simulink model "prob3"  (R2020b)
settings: Solver=ode45  StartTime=0.0  StopTime=10.0  RelTol=1e-3
undefined symbols (not defined in the file): b, m
settings Model: Creator=shridhar  LastModifiedBy=shridhar

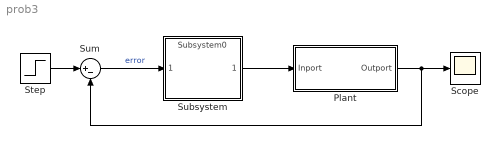
== system prob3 ==
  Plant : Subsystem
  Scope : Scope
  Step : Step  Time=0  After=u  SampleTime=0
  Subsystem : ModelReference  ModelNameDialog=Subsystem0  SimulationMode=Normal  ModelReferenceVersion=1.2
  Sum : Sum  Inputs=|+-
  wires:
  Plant/1(Outport) -> Scope/1, Sum/2
  Step/1 -> Sum/1
  Sum/1 -> Subsystem/1  "error"
  Subsystem/1 -> Plant/1(Inport)

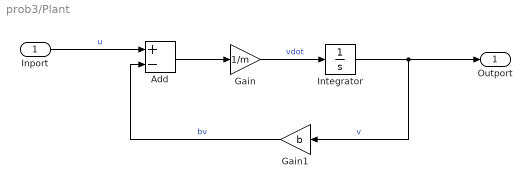
== system prob3/Plant ==
  Inport : Inport
  Add : Sum  Inputs=+-
  Gain : Gain  Gain=1/m
  Gain1 : Gain  Gain=b
  Integrator : Integrator
  Outport : Outport
  wires:
  Inport/1 -> Add/1  "u"
  Gain/1 -> Integrator/1  "vdot"
  Integrator/1 -> Gain1/1, Outport/1  "v"
  Add/1 -> Gain/1
  Gain1/1 -> Add/2  "bv"
